simulink model "motor_impedance_ctrl"  (R2023b)
settings: Solver=VariableStepAuto  StartTime=0.0  StopTime=3  FixedStep=1e-3  RelTol=1e-3
InitFcn:
  | %%%%%%%%%%%%%%%%%%%%%%%%%%%%%%%%%%%%%%%%%%%%%%%%%
  | %motor parameters
  | %we dont know these yet
  | J = 1e-6; %intertia [kg * m^2]
  | Bm = 1e-6; %kinetic friction [N * m * s]
  | 
  | %from motor datasheet
  | Km = 0.011; %motor constant (back emf constant = torque constant)
  | Rw = 1.17; %motor electric resistance in ohms
  | Lw = 0.58E-3; %motor inductance in ohms
libraries: slpidlib x1
settings Model: Creator=you29  LastModifiedBy=you29

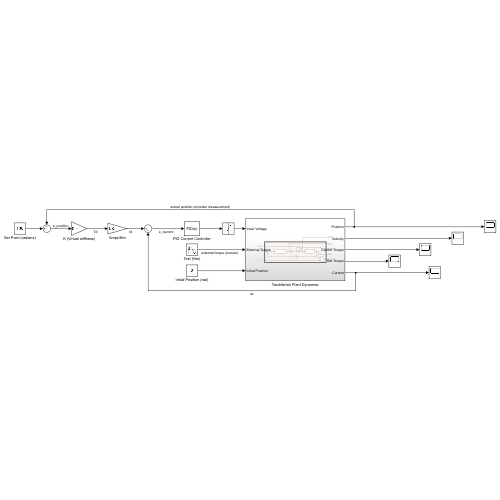
[thumbnail: Simulink's stored preview of the top-level diagram]
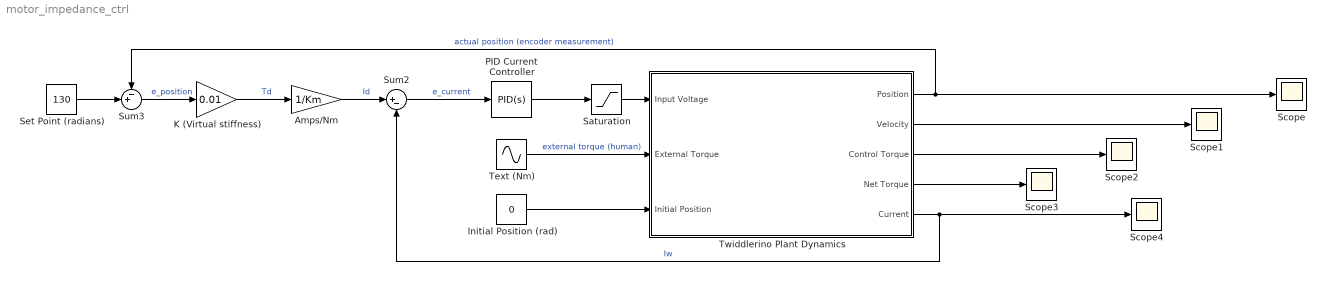
== system motor_impedance_ctrl ==
  Amps/Nm : Gain  Gain=1/Km
  Initial Position (rad) : Constant  Value=0
  K (Virtual stiffness) : Gain  Gain=0.01
  PID Current Controller : slpidlib/PID Controller  Controller=PID  Form=Parallel  TimeDomain=Continuous-time  UseExternalTs=off  SampleTime=-1  IntegratorMethod=Forward Euler  FilterMethod=Forward Euler  ControllerParametersSource=internal  P=0.36716  I=0.0056742  UseKiTs=off  D=0.18724  N=3  UseFilter=on  TunerSelectOption=Frequency Response Based  InitialConditionSource=internal  InitialConditionForIntegrator=0  InitialConditionForFilter=0  DifferentiatorICPrevScaledInput=0  ExternalReset=none  TrackingMode=off  Kt=1  LimitOutput=off  SatLimitsSource=internal  UpperSaturationLimit=inf  LowerSaturationLimit=-inf  LinearizeAsGain=on  AntiWindupMode=none  Kb=1  LimitIntegrator=off  UpperIntegratorSaturationLimit=inf  LowerIntegratorSaturationLimit=-inf  POutMin=[]  POutMax=[]  IOutMin=[]  IOutMax=[]  DOutMin=[]  DOutMax=[]  NOutMin=[]  NOutMax=[]  SumOutMin=[]  SumOutMax=[]  SaturationOutMin=[]  SaturationOutMax=[]  PParamMin=[]  PParamMax=[]  IParamMin=[]  IParamMax=[]  DParamMin=[]  DParamMax=[]  NParamMin=[]  NParamMax=[]  KbParamMin=[]  KbParamMax=[]  KtParamMin=[]  KtParamMax=[]  KbOutMin=[]  KbOutMax=[]  KtOutMin=[]  KtOutMax=[]  IntegratorOutMin=[]  IntegratorOutMax=[]  FilterOutMin=[]  FilterOutMax=[]  SumI1OutMin=[]  SumI1OutMax=[]  SumI2OutMin=[]  SumI2OutMax=[]  SumI3OutMin=[]  SumI3OutMax=[]  SumI4OutMin=[]  SumI4OutMax=[]  SumDOutMin=[]  SumDOutMax=[]  DifferentiatorOutMin=[]  DifferentiatorOutMax=[]  FilterDiffOutCoefMin=[]  FilterDiffOutCoefMax=[]  ReciprocalOutMin=[]  ReciprocalOutMax=[]  SumDenOutMin=[]  SumDenOutMax=[]  SumNumOutMin=[]  SumNumOutMax=[]  DivideOutMin=[]  DivideOutMax=[]  UdiffTsProdOutMin=[]  UdiffTsProdOutMax=[]  NTsProdOutMin=[]  NTsProdOutMax=[]  UintegralTsProdOutMin=[]  UintegralTsProdOutMax=[]  UngainTsProdOutMin=[]  UngainTsProdOutMax=[]  ClampingZeroOutDataTypeStr=Inherit: Inherit via back propagation  ClampingZeroOutMin=[]  ClampingZeroOutMax=[]  FilterDenConstantOutDataTypeStr=Inherit: Inherit via back propagation  FilterDenConstantOutMin=[]  FilterDenConstantOutMax=[]  PCopyOutDataTypeStr=Inherit: Inherit via back propagation  PCopyOutMin=[]  PCopyOutMax=[]  NCopyOutDataTypeStr=Inherit: Inherit via back propagation  NCopyOutMin=[]  NCopyOutMax=[]  IntegratorContinuousStateAttributes=''  IntegratorStateMustResolveToSignalObject=off  IntegratorRTWStateStorageClass=Auto  FilterContinuousStateAttributes=''  FilterStateMustResolveToSignalObject=off  FilterRTWStateStorageClass=Auto  ParallelPVariant=InternalParameters  IdealPVariant=Disabled  IVariant=InternalParameters  DVariant=InternalParameters  IntegratorVariant=Continuous  SatVariant=Disabled  AWVariant=Passthrough  PCopyVariant=Disabled  TRVariant=Disabled  FdbkBlocksVariant=Forward  IdealPFdbkVariant=Disabled  SatFdbkVariant=Disabled  DerivativeFilterVariant=ContFilter  NVariant=InternalParameters  NCopyVariant=Disabled  FilterICVariant=InternalICsFilter  IntegratorICVariant=InternalICs  ExternalResetVariant=Disabled  TRSumVariant=Passthrough  SumFdbkVariant=Disabled  SumVariant=Sum_PID  TsampFilterVariant=InternalTs  TsampNgainVariant=Passthrough  TsampIntegralVariant=Disabled_SignalSpec  ExternalSaturationOutDataTypeStr=Inherit: Same as second input
  Saturation : Saturate  UpperLimit=12  LowerLimit=-12  LinearizeAsGain=off
  Scope{,1..4} (5 alike) : Scope
  Set Point (radians) : Constant  Value=130
  Sum2 : Sum  Inputs=|+-
  Sum3 : Sum  Inputs=-+|
  Text (Nm) : Sin  Amplitude=1e-2  Frequency=5  SampleTime=1e-3
  Twiddlerino Plant Dynamics : Subsystem
  wires:
  Amps/Nm/1 -> Sum2/1  "Id"
  Text (Nm)/1 -> Twiddlerino Plant Dynamics/2(External Torque)  "external torque (human)"
  Sum3/1 -> K (Virtual stiffness)/1  "e_position"
  Twiddlerino Plant Dynamics/5(Current) -> Sum2/2, Scope4/1  "Iw"
  Twiddlerino Plant Dynamics/1(Position) -> Sum3/1, Scope/1  "actual position (encoder measurement)"
  Initial Position (rad)/1 -> Twiddlerino Plant Dynamics/3(Initial Position)
  K (Virtual stiffness)/1 -> Amps/Nm/1  "Td"
  Twiddlerino Plant Dynamics/3(Control Torque) -> Scope2/1
  Saturation/1 -> Twiddlerino Plant Dynamics/1(Input Voltage)
  Twiddlerino Plant Dynamics/2(Velocity) -> Scope1/1
  Sum2/1 -> PID Current Controller/1  "e_current"
  PID Current Controller/1 -> Saturation/1
  Twiddlerino Plant Dynamics/4(Net Torque) -> Scope3/1
  Set Point (radians)/1 -> Sum3/2

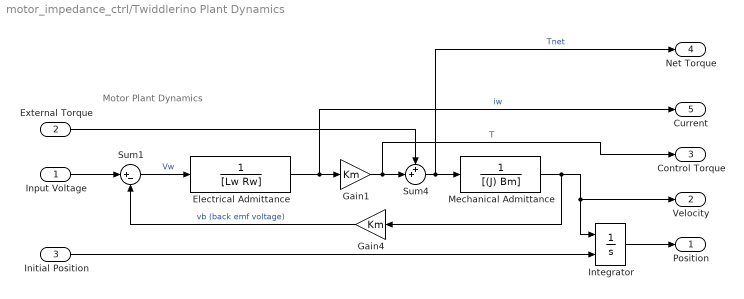
== system motor_impedance_ctrl/Twiddlerino Plant Dynamics ==
  note: Motor Plant Dynamics
  Input Voltage : Inport
  External Torque : Inport  Port=2
  Initial Position : Inport  Port=3
  Electrical Admittance : TransferFcn  Denominator=[Lw Rw]
  Gain1 : Gain  Gain=Km
  Gain4 : Gain  Gain=Km
  Integrator : Integrator  InitialConditionSource=external
  Mechanical Admittance : TransferFcn  Denominator=[(J) Bm]
  Sum1 : Sum  Inputs=|+-
  Sum4 : Sum  Inputs=++|
  Position : Outport
  Velocity : Outport  Port=2
  Control Torque : Outport  Port=3
  Net Torque : Outport  Port=4
  Current : Outport  Port=5
  wires:
  Integrator/1 -> Position/1
  Gain1/1 -> Control Torque/1, Sum4/2  "T"
  External Torque/1 -> Sum4/1
  Electrical Admittance/1 -> Current/1, Gain1/1  "iw"
  Initial Position/1 -> Integrator/2
  Mechanical Admittance/1 -> Gain4/1, Integrator/1, Velocity/1
  Sum4/1 -> Net Torque/1, Mechanical Admittance/1  "Tnet"
  Gain4/1 -> Sum1/2  "vb (back emf voltage)"
  Input Voltage/1 -> Sum1/1
  Sum1/1 -> Electrical Admittance/1  "Vw"
